simulink model "MdXX_Status"  (R2018b)
settings: Solver=FixedStepDiscrete  StartTime=0.0  StopTime=10.0  FixedStep=0.01  RelTol=1e-3
undefined symbols (not defined in the file or in its folder): data, NvStMdxxMemStatusKam_Set
libraries: RspLib x94, simulink x1
(part 2 of 2)

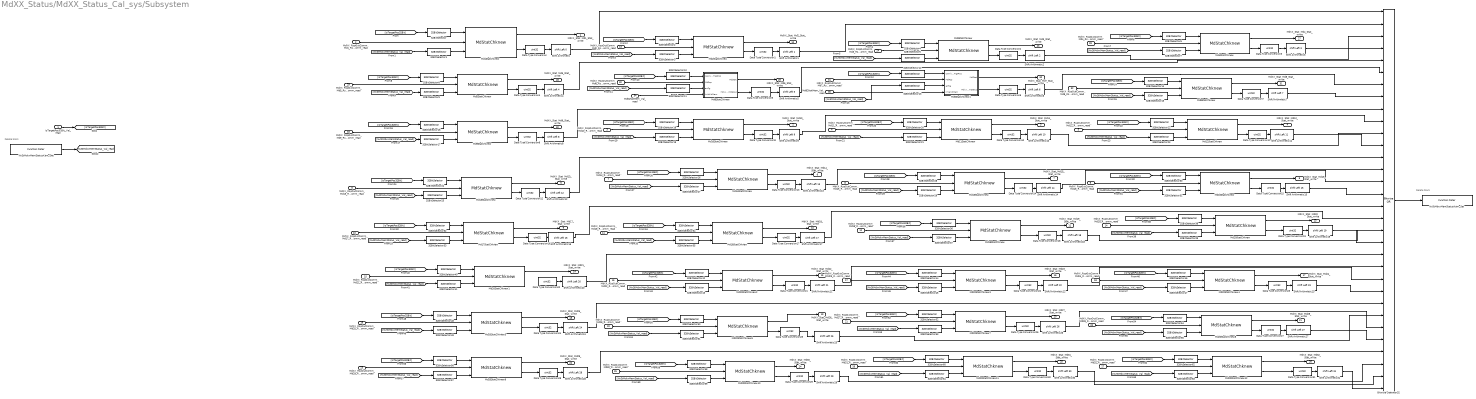
== system MdXX_Status/MdXX_Status_Cal_sys/Subsystem ==
  note: Delete block
  note: Delete block
  IsTargetPos32Bit_Val_read : Inport
  MdXX_RspOutComm_Md1_RspOutComm_read : Inport  Port=2
  MdXX_RspOutComm_Md10_RspOutComm_read : Inport  Port=3
  MdXX_RspOutComm_Md11_RspOutComm_read : Inport  Port=4
  MdXX_RspOutComm_Md12_RspOutComm_read : Inport  Port=5
  MdXX_RspOutComm_Md13_RspOutComm_read : Inport  Port=6
  MdXX_RspOutComm_Md14_RspOutComm_read : Inport  Port=7
  MdXX_RspOutComm_Md15_RspOutComm_read : Inport  Port=8
  MdXX_RspOutComm_Md16_RspOutComm_read : Inport  Port=9
  MdXX_RspOutComm_Md17_RspOutComm_read : Inport  Port=10
  MdXX_RspOutComm_Md18_RspOutComm_read : Inport  Port=11
  MdXX_RspOutComm_Md19_RspOutComm_read : Inport  Port=12
  MdXX_RspOutComm_Md2_RspOutComm_read : Inport  Port=13
  MdXX_RspOutComm_Md20_RspOutComm_read : Inport  Port=14
  MdXX_RspOutComm_Md21_RspOutComm_read : Inport  Port=15
  MdXX_RspOutComm_Md22_RspOutComm_read : Inport  Port=16
  MdXX_RspOutComm_Md23_RspOutComm_read : Inport  Port=17
  MdXX_RspOutComm_Md24_RspOutComm_read : Inport  Port=18
  MdXX_RspOutComm_Md25_RspOutComm_read : Inport  Port=19
  MdXX_RspOutComm_Md26_RspOutComm_read : Inport  Port=20
  MdXX_RspOutComm_Md27_RspOutComm_read : Inport  Port=21
  MdXX_RspOutComm_Md28_RspOutComm_read : Inport  Port=22
  MdXX_RspOutComm_Md29_RspOutComm_read : Inport  Port=23
  MdXX_RspOutComm_Md3_RspOutComm_read : Inport  Port=24
  MdXX_RspOutComm_Md30_RspOutComm_read : Inport  Port=25
  MdXX_RspOutComm_Md31_RspOutComm_read : Inport  Port=26
  MdXX_RspOutComm_Md32_RspOutComm_read : Inport  Port=27
  MdXX_RspOutComm_Md4_RspOutComm_read : Inport  Port=28
  MdXX_RspOutComm_Md5_RspOutComm_read : Inport  Port=29
  MdXX_RspOutComm_Md6_RspOutComm_read : Inport  Port=30
  MdXX_RspOutComm_Md7_RspOutComm_read : Inport  Port=31
  MdXX_RspOutComm_Md8_RspOutComm_read : Inport  Port=32
  MdXX_RspOutComm_Md9_RspOutComm_read : Inport  Port=33
  Md61NotMem_Val_read : Inport  Port=34
  Md62NotMem_Val_read : Inport  Port=35
  32BitSelector : RspLib/32BitSelector  BitNum=0
  32BitSelector1 : RspLib/32BitSelector  BitNum=0
  32BitSelector10 : RspLib/32BitSelector  BitNum=5
  32BitSelector11 : RspLib/32BitSelector  BitNum=5
  32BitSelector12 : RspLib/32BitSelector  BitNum=6
  32BitSelector13 : RspLib/32BitSelector  BitNum=6
  32BitSelector14 : RspLib/32BitSelector  BitNum=7
  32BitSelector15 : RspLib/32BitSelector  BitNum=7
  32BitSelector16 : RspLib/32BitSelector  BitNum=8
  32BitSelector17 : RspLib/32BitSelector  BitNum=8
  32BitSelector18 : RspLib/32BitSelector  BitNum=9
  32BitSelector19 : RspLib/32BitSelector  BitNum=9
  32BitSelector2 : RspLib/32BitSelector  BitNum=1
  32BitSelector20 : RspLib/32BitSelector  BitNum=10
  32BitSelector21 : RspLib/32BitSelector  BitNum=10
  32BitSelector22 : RspLib/32BitSelector  BitNum=11
  32BitSelector23 : RspLib/32BitSelector  BitNum=11
  32BitSelector24 : RspLib/32BitSelector  BitNum=12
  32BitSelector25 : RspLib/32BitSelector  BitNum=12
  32BitSelector26 : RspLib/32BitSelector  BitNum=13
  32BitSelector27 : RspLib/32BitSelector  BitNum=13
  32BitSelector28 : RspLib/32BitSelector  BitNum=14
  32BitSelector29 : RspLib/32BitSelector  BitNum=14
  32BitSelector3 : RspLib/32BitSelector  BitNum=1
  32BitSelector30 : RspLib/32BitSelector  BitNum=15
  32BitSelector31 : RspLib/32BitSelector  BitNum=15
  32BitSelector32 : RspLib/32BitSelector  BitNum=16
  32BitSelector33 : RspLib/32BitSelector  BitNum=16
  32BitSelector34 : RspLib/32BitSelector  BitNum=17
  32BitSelector35 : RspLib/32BitSelector  BitNum=17
  32BitSelector36 : RspLib/32BitSelector  BitNum=18
  32BitSelector37 : RspLib/32BitSelector  BitNum=18
  32BitSelector38 : RspLib/32BitSelector  BitNum=19
  32BitSelector39 : RspLib/32BitSelector  BitNum=19
  32BitSelector4 : RspLib/32BitSelector  BitNum=2
  32BitSelector40 : RspLib/32BitSelector  BitNum=20
  32BitSelector41 : RspLib/32BitSelector  BitNum=20
  32BitSelector42 : RspLib/32BitSelector  BitNum=21
  32BitSelector43 : RspLib/32BitSelector  BitNum=21
  32BitSelector44 : RspLib/32BitSelector  BitNum=22
  32BitSelector45 : RspLib/32BitSelector  BitNum=22
  32BitSelector46 : RspLib/32BitSelector  BitNum=23
  32BitSelector47 : RspLib/32BitSelector  BitNum=23
  32BitSelector48 : RspLib/32BitSelector  BitNum=24
  32BitSelector49 : RspLib/32BitSelector  BitNum=24
  32BitSelector5 : RspLib/32BitSelector  BitNum=2
  32BitSelector50 : RspLib/32BitSelector  BitNum=25
  32BitSelector51 : RspLib/32BitSelector  BitNum=25
  32BitSelector52 : RspLib/32BitSelector  BitNum=26
  32BitSelector53 : RspLib/32BitSelector  BitNum=26
  32BitSelector54 : RspLib/32BitSelector  BitNum=27
  32BitSelector55 : RspLib/32BitSelector  BitNum=27
  32BitSelector56 : RspLib/32BitSelector  BitNum=28
  32BitSelector57 : RspLib/32BitSelector  BitNum=28
  32BitSelector58 : RspLib/32BitSelector  BitNum=29
  32BitSelector59 : RspLib/32BitSelector  BitNum=29
  32BitSelector6 : RspLib/32BitSelector  BitNum=3
  32BitSelector60 : RspLib/32BitSelector  BitNum=30
  32BitSelector61 : RspLib/32BitSelector  BitNum=30
  32BitSelector62 : RspLib/32BitSelector  BitNum=31
  32BitSelector63 : RspLib/32BitSelector  BitNum=31
  32BitSelector7 : RspLib/32BitSelector  BitNum=3
  32BitSelector8 : RspLib/32BitSelector  BitNum=4
  32BitSelector9 : RspLib/32BitSelector  BitNum=4
  Bitwise Operator32 : simulink/Logic and Bit Operations/Bitwise Operator  logicop=OR  UseBitMask=off  NumInputPorts=32  BitMask=bin2dec('11011001')  BitMaskRealWorld=Stored Integer
  Data Type Conversion{,1..31} (32 alike) : DataTypeConversion  OutDataTypeStr=uint32
  Md10StatChknew : RspLib/MdStatChknew  SystemSampleTime=-1
  Md11StatChknew : RspLib/MdStatChknew  SystemSampleTime=-1
  Md12StatChknew : RspLib/MdStatChknew  SystemSampleTime=-1
  Md13StatChknew : RspLib/MdStatChknew  SystemSampleTime=-1
  Md14StatChknew : RspLib/MdStatChknew  SystemSampleTime=-1
  Md15StatChknew : RspLib/MdStatChknew  SystemSampleTime=-1
  Md16StatChknew : RspLib/MdStatChknew  SystemSampleTime=-1
  Md17StatChknew : RspLib/MdStatChknew  SystemSampleTime=-1
  Md18StatChknew : RspLib/MdStatChknew  SystemSampleTime=-1
  Md19StatChknew : RspLib/MdStatChknew  SystemSampleTime=-1
  Md1StatChknew : RspLib/MdStatChknew  SystemSampleTime=-1
  Md20StatChknew{,1..12} (13 alike) : RspLib/MdStatChknew  SystemSampleTime=-1
  Md2StatChknew : RspLib/MdStatChknew  SystemSampleTime=-1
  Md3StatChknew : RspLib/MdStatChknew  SystemSampleTime=-1
  Md4StatChknew : RspLib/MdStatChknew  SystemSampleTime=-1
  Md5StatChknew : RspLib/MdStatChknew  SystemSampleTime=-1
  Md6StatChknew : Subsystem
  Md6StatChknew1 : Subsystem
  Md8StatChknew : RspLib/MdStatChknew  SystemSampleTime=-1
  Md9StatChknew : RspLib/MdStatChknew  SystemSampleTime=-1
  NvStMdxxMemStatusKam_Get : FunctionCaller  FunctionPrototype=data = NvStMdxxMemStatusKam_Get()  OutputArgumentSpecifications=uint32(1)
  NvStMdxxMemStatusKam_Set : FunctionCaller  FunctionPrototype=NvStMdxxMemStatusKam_Set(data)  InputArgumentSpecifications=uint32(1)
  Shift Arithmetic : ArithShift  BitShiftDirection=Left
  Shift Arithmetic1 : ArithShift  BitShiftNumber=1  BitShiftDirection=Left
  Shift Arithmetic10 : ArithShift  BitShiftNumber=10  BitShiftDirection=Left
  Shift Arithmetic11 : ArithShift  BitShiftNumber=11  BitShiftDirection=Left
  Shift Arithmetic12 : ArithShift  BitShiftNumber=12  BitShiftDirection=Left
  Shift Arithmetic13 : ArithShift  BitShiftNumber=13  BitShiftDirection=Left
  Shift Arithmetic14 : ArithShift  BitShiftNumber=14  BitShiftDirection=Left
  Shift Arithmetic15 : ArithShift  BitShiftNumber=15  BitShiftDirection=Left
  Shift Arithmetic16 : ArithShift  BitShiftNumber=16  BitShiftDirection=Left
  Shift Arithmetic17 : ArithShift  BitShiftNumber=17  BitShiftDirection=Left
  Shift Arithmetic18 : ArithShift  BitShiftNumber=18  BitShiftDirection=Left
  Shift Arithmetic19 : ArithShift  BitShiftNumber=19  BitShiftDirection=Left
  Shift Arithmetic2 : ArithShift  BitShiftNumber=2  BitShiftDirection=Left
  Shift Arithmetic20 : ArithShift  BitShiftNumber=20  BitShiftDirection=Left
  Shift Arithmetic21 : ArithShift  BitShiftNumber=21  BitShiftDirection=Left
  Shift Arithmetic22 : ArithShift  BitShiftNumber=22  BitShiftDirection=Left
  Shift Arithmetic23 : ArithShift  BitShiftNumber=23  BitShiftDirection=Left
  Shift Arithmetic24 : ArithShift  BitShiftNumber=24  BitShiftDirection=Left
  Shift Arithmetic25 : ArithShift  BitShiftNumber=25  BitShiftDirection=Left
  Shift Arithmetic26 : ArithShift  BitShiftNumber=26  BitShiftDirection=Left
  Shift Arithmetic27 : ArithShift  BitShiftNumber=27  BitShiftDirection=Left
  Shift Arithmetic28 : ArithShift  BitShiftNumber=28  BitShiftDirection=Left
  Shift Arithmetic29 : ArithShift  BitShiftNumber=29  BitShiftDirection=Left
  Shift Arithmetic3 : ArithShift  BitShiftNumber=3  BitShiftDirection=Left
  Shift Arithmetic30 : ArithShift  BitShiftNumber=30  BitShiftDirection=Left
  Shift Arithmetic31 : ArithShift  BitShiftNumber=31  BitShiftDirection=Left
  Shift Arithmetic4 : ArithShift  BitShiftNumber=4  BitShiftDirection=Left
  Shift Arithmetic5 : ArithShift  BitShiftNumber=5  BitShiftDirection=Left
  Shift Arithmetic6 : ArithShift  BitShiftNumber=6  BitShiftDirection=Left
  Shift Arithmetic7 : ArithShift  BitShiftNumber=7  BitShiftDirection=Left
  Shift Arithmetic8 : ArithShift  BitShiftNumber=8  BitShiftDirection=Left
  Shift Arithmetic9 : ArithShift  BitShiftNumber=9  BitShiftDirection=Left
  MdXX_Stat_Md1_Stat_write : Outport
      settings: EnsureOutportIsVirtual=on
  MdXX_Stat_Md10_Stat_write : Outport  Port=2
      settings: EnsureOutportIsVirtual=on
  MdXX_Stat_Md11_Stat_write : Outport  Port=3
      settings: EnsureOutportIsVirtual=on
  MdXX_Stat_Md12_Stat_write : Outport  Port=4
      settings: EnsureOutportIsVirtual=on
  MdXX_Stat_Md13_Stat_write : Outport  Port=5
      settings: EnsureOutportIsVirtual=on
  MdXX_Stat_Md14_Stat_write : Outport  Port=6
      settings: EnsureOutportIsVirtual=on
  MdXX_Stat_Md15_Stat_write : Outport  Port=7
      settings: EnsureOutportIsVirtual=on
  MdXX_Stat_Md16_Stat_write : Outport  Port=8
      settings: EnsureOutportIsVirtual=on
  MdXX_Stat_Md17_Stat_write : Outport  Port=9
      settings: EnsureOutportIsVirtual=on
  MdXX_Stat_Md18_Stat_write : Outport  Port=10
      settings: EnsureOutportIsVirtual=on
  MdXX_Stat_Md19_Stat_write : Outport  Port=11
      settings: EnsureOutportIsVirtual=on
  MdXX_Stat_Md2_Stat_write : Outport  Port=12
      settings: EnsureOutportIsVirtual=on
  MdXX_Stat_Md20_Stat_write : Outport  Port=13
      settings: EnsureOutportIsVirtual=on
  MdXX_Stat_Md21_Stat_write : Outport  Port=14
      settings: EnsureOutportIsVirtual=on
  MdXX_Stat_Md22_Stat_write : Outport  Port=15
      settings: EnsureOutportIsVirtual=on
  MdXX_Stat_Md23_Stat_write : Outport  Port=16
      settings: EnsureOutportIsVirtual=on
  MdXX_Stat_Md24_Stat_write : Outport  Port=17
      settings: EnsureOutportIsVirtual=on
  MdXX_Stat_Md25_Stat_write : Outport  Port=18
      settings: EnsureOutportIsVirtual=on
  MdXX_Stat_Md26_Stat_write : Outport  Port=19
      settings: EnsureOutportIsVirtual=on
  MdXX_Stat_Md27_Stat_write : Outport  Port=20
      settings: EnsureOutportIsVirtual=on
  MdXX_Stat_Md28_Stat_write : Outport  Port=21
      settings: EnsureOutportIsVirtual=on
  MdXX_Stat_Md29_Stat_write : Outport  Port=22
      settings: EnsureOutportIsVirtual=on
  MdXX_Stat_Md3_Stat_write : Outport  Port=23
      settings: EnsureOutportIsVirtual=on
  MdXX_Stat_Md30_Stat_write : Outport  Port=24
      settings: EnsureOutportIsVirtual=on
  MdXX_Stat_Md31_Stat_write : Outport  Port=25
      settings: EnsureOutportIsVirtual=on
  MdXX_Stat_Md32_Stat_write : Outport  Port=26
      settings: EnsureOutportIsVirtual=on
  MdXX_Stat_Md4_Stat_write : Outport  Port=27
      settings: EnsureOutportIsVirtual=on
  MdXX_Stat_Md5_Stat_write : Outport  Port=28
      settings: EnsureOutportIsVirtual=on
  MdXX_Stat_Md6_Stat_write : Outport  Port=29
      settings: EnsureOutportIsVirtual=on
  MdXX_Stat_Md7_Stat_write : Outport  Port=30
      settings: EnsureOutportIsVirtual=on
  MdXX_Stat_Md8_Stat_write : Outport  Port=31
      settings: EnsureOutportIsVirtual=on
  MdXX_Stat_Md9_Stat_write : Outport  Port=32
      settings: EnsureOutportIsVirtual=on
  wires:
  IsTargetPos32Bit_Val_read/1 -> [IsTargetPos32Bit]
  [IsTargetPos32Bit] -> 32BitSelector/1
  32BitSelector/1 -> Md1StatChknew/1
  32BitSelector1/1 -> Md1StatChknew/3
  MdXX_RspOutComm_Md1_RspOutComm_read/1 -> Md1StatChknew/2
  MdXX_RspOutComm_Md2_RspOutComm_read/1 -> Md2StatChknew/2
  32BitSelector3/1 -> Md2StatChknew/3
  32BitSelector2/1 -> Md2StatChknew/1
  [IsTargetPos32Bit] -> 32BitSelector2/1
  [NvStMdxxMemStatus_Val_read] -> 32BitSelector5/1
  [IsTargetPos32Bit] -> 32BitSelector4/1
  32BitSelector4/1 -> Md3StatChknew/1
  32BitSelector5/1 -> Md3StatChknew/3
  MdXX_RspOutComm_Md3_RspOutComm_read/1 -> Md3StatChknew/2
  MdXX_RspOutComm_Md4_RspOutComm_read/1 -> Md4StatChknew/2
  32BitSelector7/1 -> Md4StatChknew/3
  32BitSelector6/1 -> Md4StatChknew/1
  [IsTargetPos32Bit] -> 32BitSelector6/1
  [NvStMdxxMemStatus_Val_read] -> 32BitSelector7/1
  [IsTargetPos32Bit] -> 32BitSelector8/1
  32BitSelector8/1 -> Md5StatChknew/1
  32BitSelector9/1 -> Md5StatChknew/3
  MdXX_RspOutComm_Md5_RspOutComm_read/1 -> Md5StatChknew/2
  MdXX_RspOutComm_Md6_RspOutComm_read/1 -> Md6StatChknew/2(MdRsp)
  32BitSelector11/1 -> Md6StatChknew/3(enflg)
  32BitSelector10/1 -> Md6StatChknew/1(IsArrivedTrgtPos)
  [IsTargetPos32Bit] -> 32BitSelector10/1
  [NvStMdxxMemStatus_Val_read] -> 32BitSelector11/1
  [IsTargetPos32Bit] -> 32BitSelector12/1
  32BitSelector12/1 -> Md6StatChknew1/1(IsArrivedTrgtPos)
  32BitSelector13/1 -> Md6StatChknew1/3(enflg)
  MdXX_RspOutComm_Md7_RspOutComm_read/1 -> Md6StatChknew1/2(MdRsp)
  MdXX_RspOutComm_Md8_RspOutComm_read/1 -> Md8StatChknew/2
  32BitSelector15/1 -> Md8StatChknew/3
  32BitSelector14/1 -> Md8StatChknew/1
  [IsTargetPos32Bit] -> 32BitSelector14/1
  [IsTargetPos32Bit] -> 32BitSelector16/1
  32BitSelector16/1 -> Md9StatChknew/1
  32BitSelector17/1 -> Md9StatChknew/3
  MdXX_RspOutComm_Md9_RspOutComm_read/1 -> Md9StatChknew/2
  MdXX_RspOutComm_Md10_RspOutComm_read/1 -> Md10StatChknew/2
  32BitSelector19/1 -> Md10StatChknew/3
  32BitSelector18/1 -> Md10StatChknew/1
  [IsTargetPos32Bit] -> 32BitSelector18/1
  [IsTargetPos32Bit] -> 32BitSelector20/1
  32BitSelector20/1 -> Md11StatChknew/1
  32BitSelector21/1 -> Md11StatChknew/3
  MdXX_RspOutComm_Md11_RspOutComm_read/1 -> Md11StatChknew/2
  MdXX_RspOutComm_Md12_RspOutComm_read/1 -> Md12StatChknew/2
  32BitSelector23/1 -> Md12StatChknew/3
  32BitSelector22/1 -> Md12StatChknew/1
  [IsTargetPos32Bit] -> 32BitSelector22/1
  [IsTargetPos32Bit] -> 32BitSelector24/1
  32BitSelector24/1 -> Md13StatChknew/1
  32BitSelector25/1 -> Md13StatChknew/3
  MdXX_RspOutComm_Md13_RspOutComm_read/1 -> Md13StatChknew/2
  MdXX_RspOutComm_Md14_RspOutComm_read/1 -> Md14StatChknew/2
  32BitSelector27/1 -> Md14StatChknew/3
  32BitSelector26/1 -> Md14StatChknew/1
  [IsTargetPos32Bit] -> 32BitSelector26/1
  [IsTargetPos32Bit] -> 32BitSelector28/1
  32BitSelector28/1 -> Md15StatChknew/1
  32BitSelector29/1 -> Md15StatChknew/3
  MdXX_RspOutComm_Md15_RspOutComm_read/1 -> Md15StatChknew/2
  MdXX_RspOutComm_Md16_RspOutComm_read/1 -> Md16StatChknew/2
  32BitSelector31/1 -> Md16StatChknew/3
  32BitSelector30/1 -> Md16StatChknew/1
  [IsTargetPos32Bit] -> 32BitSelector30/1
  [IsTargetPos32Bit] -> 32BitSelector32/1
  32BitSelector32/1 -> Md17StatChknew/1
  32BitSelector33/1 -> Md17StatChknew/3
  MdXX_RspOutComm_Md17_RspOutComm_read/1 -> Md17StatChknew/2
  MdXX_RspOutComm_Md18_RspOutComm_read/1 -> Md18StatChknew/2
  32BitSelector35/1 -> Md18StatChknew/3
  32BitSelector34/1 -> Md18StatChknew/1
  [IsTargetPos32Bit] -> 32BitSelector34/1
  [IsTargetPos32Bit] -> 32BitSelector36/1
  32BitSelector36/1 -> Md19StatChknew/1
  32BitSelector37/1 -> Md19StatChknew/3
  MdXX_RspOutComm_Md19_RspOutComm_read/1 -> Md19StatChknew/2
  MdXX_RspOutComm_Md20_RspOutComm_read/1 -> Md20StatChknew/2
  32BitSelector39/1 -> Md20StatChknew/3
  32BitSelector38/1 -> Md20StatChknew/1
  [IsTargetPos32Bit] -> 32BitSelector38/1
  Md1StatChknew/1 -> MdXX_Stat_Md1_Stat_write/1
  Md2StatChknew/1 -> MdXX_Stat_Md2_Stat_write/1
  Md3StatChknew/1 -> MdXX_Stat_Md3_Stat_write/1
  Md4StatChknew/1 -> MdXX_Stat_Md4_Stat_write/1
  Md5StatChknew/1 -> MdXX_Stat_Md5_Stat_write/1
  Md6StatChknew/1(MdStat) -> MdXX_Stat_Md6_Stat_write/1
  Md6StatChknew1/1(MdStat) -> MdXX_Stat_Md7_Stat_write/1
  Md8StatChknew/1 -> MdXX_Stat_Md8_Stat_write/1
  Md9StatChknew/1 -> MdXX_Stat_Md9_Stat_write/1
  Md10StatChknew/1 -> MdXX_Stat_Md10_Stat_write/1
  Md11StatChknew/1 -> MdXX_Stat_Md11_Stat_write/1
  Md12StatChknew/1 -> MdXX_Stat_Md12_Stat_write/1
  Md13StatChknew/1 -> MdXX_Stat_Md13_Stat_write/1
  Md14StatChknew/1 -> MdXX_Stat_Md14_Stat_write/1
  Md15StatChknew/1 -> MdXX_Stat_Md15_Stat_write/1
  Md16StatChknew/1 -> MdXX_Stat_Md16_Stat_write/1
  Md17StatChknew/1 -> MdXX_Stat_Md17_Stat_write/1
  Md18StatChknew/1 -> MdXX_Stat_Md18_Stat_write/1
  Md19StatChknew/1 -> MdXX_Stat_Md19_Stat_write/1
  Md20StatChknew/1 -> MdXX_Stat_Md20_Stat_write/1
  Md20StatChknew1/1 -> MdXX_Stat_Md21_Stat_write/1
  [IsTargetPos32Bit] -> 32BitSelector40/1
  32BitSelector40/1 -> Md20StatChknew1/1
  32BitSelector41/1 -> Md20StatChknew1/3
  MdXX_RspOutComm_Md21_RspOutComm_read/1 -> Md20StatChknew1/2
  MdXX_RspOutComm_Md22_RspOutComm_read/1 -> Md20StatChknew2/2
  32BitSelector43/1 -> Md20StatChknew2/3
  32BitSelector42/1 -> Md20StatChknew2/1
  [IsTargetPos32Bit] -> 32BitSelector42/1
  Md20StatChknew2/1 -> MdXX_Stat_Md22_Stat_write/1
  Md20StatChknew3/1 -> MdXX_Stat_Md23_Stat_write/1
  [IsTargetPos32Bit] -> 32BitSelector44/1
  32BitSelector44/1 -> Md20StatChknew3/1
  32BitSelector45/1 -> Md20StatChknew3/3
  MdXX_RspOutComm_Md23_RspOutComm_read/1 -> Md20StatChknew3/2
  MdXX_RspOutComm_Md24_RspOutComm_read/1 -> Md20StatChknew4/2
  32BitSelector47/1 -> Md20StatChknew4/3
  32BitSelector46/1 -> Md20StatChknew4/1
  [IsTargetPos32Bit] -> 32BitSelector46/1
  Md20StatChknew4/1 -> MdXX_Stat_Md24_Stat_write/1
  Md20StatChknew5/1 -> MdXX_Stat_Md25_Stat_write/1
  [IsTargetPos32Bit] -> 32BitSelector48/1
  32BitSelector48/1 -> Md20StatChknew5/1
  32BitSelector49/1 -> Md20StatChknew5/3
  MdXX_RspOutComm_Md25_RspOutComm_read/1 -> Md20StatChknew5/2
  MdXX_RspOutComm_Md26_RspOutComm_read/1 -> Md20StatChknew6/2
  32BitSelector51/1 -> Md20StatChknew6/3
  32BitSelector50/1 -> Md20StatChknew6/1
  [IsTargetPos32Bit] -> 32BitSelector50/1
  Md20StatChknew6/1 -> MdXX_Stat_Md26_Stat_write/1
  Md20StatChknew7/1 -> MdXX_Stat_Md27_Stat_write/1
  [IsTargetPos32Bit] -> 32BitSelector52/1
  32BitSelector52/1 -> Md20StatChknew7/1
  32BitSelector53/1 -> Md20StatChknew7/3
  MdXX_RspOutComm_Md27_RspOutComm_read/1 -> Md20StatChknew7/2
  MdXX_RspOutComm_Md28_RspOutComm_read/1 -> Md20StatChknew8/2
  32BitSelector55/1 -> Md20StatChknew8/3
  32BitSelector54/1 -> Md20StatChknew8/1
  [IsTargetPos32Bit] -> 32BitSelector54/1
  Md20StatChknew8/1 -> MdXX_Stat_Md28_Stat_write/1
  Md20StatChknew9/1 -> MdXX_Stat_Md29_Stat_write/1
  [IsTargetPos32Bit] -> 32BitSelector56/1
  32BitSelector56/1 -> Md20StatChknew9/1
  32BitSelector57/1 -> Md20StatChknew9/3
  MdXX_RspOutComm_Md29_RspOutComm_read/1 -> Md20StatChknew9/2
  MdXX_RspOutComm_Md30_RspOutComm_read/1 -> Md20StatChknew10/2
  32BitSelector59/1 -> Md20StatChknew10/3
  32BitSelector58/1 -> Md20StatChknew10/1
  [IsTargetPos32Bit] -> 32BitSelector58/1
  Md20StatChknew10/1 -> MdXX_Stat_Md30_Stat_write/1
  Md20StatChknew11/1 -> MdXX_Stat_Md31_Stat_write/1
  [IsTargetPos32Bit] -> 32BitSelector60/1
  32BitSelector60/1 -> Md20StatChknew11/1
  32BitSelector61/1 -> Md20StatChknew11/3
  MdXX_RspOutComm_Md31_RspOutComm_read/1 -> Md20StatChknew11/2
  MdXX_RspOutComm_Md32_RspOutComm_read/1 -> Md20StatChknew12/2
  32BitSelector63/1 -> Md20StatChknew12/3
  32BitSelector62/1 -> Md20StatChknew12/1
  [IsTargetPos32Bit] -> 32BitSelector62/1
  Md20StatChknew12/1 -> MdXX_Stat_Md32_Stat_write/1
  Md61NotMem_Val_read/1 -> Md6StatChknew/4(InValidMem)
  Md62NotMem_Val_read/1 -> Md6StatChknew1/4(InValidMem)
  Data Type Conversion/1 -> Shift Arithmetic/1
  Md1StatChknew/2 -> Data Type Conversion/1
  Shift Arithmetic/1 -> Bitwise Operator32/1
  [NvStMdxxMemStatus_Val_read] -> 32BitSelector1/1
  Md2StatChknew/2 -> Data Type Conversion1/1
  [NvStMdxxMemStatus_Val_read] -> 32BitSelector3/1
  Data Type Conversion1/1 -> Shift Arithmetic1/1
  Shift Arithmetic1/1 -> Bitwise Operator32/2
  Md3StatChknew/2 -> Data Type Conversion2/1
  Data Type Conversion2/1 -> Shift Arithmetic2/1
  Shift Arithmetic2/1 -> Bitwise Operator32/3
  Md4StatChknew/2 -> Data Type Conversion3/1
  Data Type Conversion3/1 -> Shift Arithmetic3/1
  Shift Arithmetic3/1 -> Bitwise Operator32/4
  Md5StatChknew/2 -> Data Type Conversion4/1
  Data Type Conversion4/1 -> Shift Arithmetic4/1
  Shift Arithmetic4/1 -> Bitwise Operator32/5
  Md6StatChknew/2(MdxxMemStatus) -> Data Type Conversion5/1
  Data Type Conversion5/1 -> Shift Arithmetic5/1
  Md6StatChknew1/2(MdxxMemStatus) -> Data Type Conversion6/1
  [NvStMdxxMemStatus_Val_read] -> 32BitSelector13/1
  Data Type Conversion6/1 -> Shift Arithmetic6/1
  Md8StatChknew/2 -> Data Type Conversion7/1
  Data Type Conversion7/1 -> Shift Arithmetic7/1
  Shift Arithmetic7/1 -> Bitwise Operator32/8
  Md9StatChknew/2 -> Data Type Conversion8/1
  Data Type Conversion8/1 -> Shift Arithmetic8/1
  Shift Arithmetic8/1 -> Bitwise Operator32/9
  Md10StatChknew/2 -> Data Type Conversion9/1
  Data Type Conversion9/1 -> Shift Arithmetic9/1
  Shift Arithmetic9/1 -> Bitwise Operator32/10
  Md11StatChknew/2 -> Data Type Conversion10/1
  Data Type Conversion10/1 -> Shift Arithmetic10/1
  Shift Arithmetic10/1 -> Bitwise Operator32/11
  [NvStMdxxMemStatus_Val_read] -> 32BitSelector21/1
  Md12StatChknew/2 -> Data Type Conversion11/1
  Data Type Conversion11/1 -> Shift Arithmetic11/1
  Shift Arithmetic11/1 -> Bitwise Operator32/12
  Md13StatChknew/2 -> Data Type Conversion12/1
  Data Type Conversion12/1 -> Shift Arithmetic12/1
  Shift Arithmetic12/1 -> Bitwise Operator32/13
  Md14StatChknew/2 -> Data Type Conversion13/1
  Data Type Conversion13/1 -> Shift Arithmetic13/1
  Shift Arithmetic13/1 -> Bitwise Operator32/14
  Shift Arithmetic14/1 -> Bitwise Operator32/15
  Data Type Conversion14/1 -> Shift Arithmetic14/1
  Md15StatChknew/2 -> Data Type Conversion14/1
  Shift Arithmetic15/1 -> Bitwise Operator32/16
  Data Type Conversion15/1 -> Shift Arithmetic15/1
  Md16StatChknew/2 -> Data Type Conversion15/1
  Shift Arithmetic16/1 -> Bitwise Operator32/17
  Data Type Conversion16/1 -> Shift Arithmetic16/1
  Md17StatChknew/2 -> Data Type Conversion16/1
  Shift Arithmetic17/1 -> Bitwise Operator32/18
  Data Type Conversion17/1 -> Shift Arithmetic17/1
  Md18StatChknew/2 -> Data Type Conversion17/1
  Shift Arithmetic18/1 -> Bitwise Operator32/19
  Data Type Conversion18/1 -> Shift Arithmetic18/1
  Md19StatChknew/2 -> Data Type Conversion18/1
  Shift Arithmetic19/1 -> Bitwise Operator32/20
  Data Type Conversion19/1 -> Shift Arithmetic19/1
  Md20StatChknew/2 -> Data Type Conversion19/1
  Shift Arithmetic20/1 -> Bitwise Operator32/21
  Data Type Conversion20/1 -> Shift Arithmetic20/1
  ? -> Data Type Conversion20/1
  Shift Arithmetic21/1 -> Bitwise Operator32/22
  Data Type Conversion21/1 -> Shift Arithmetic21/1
  Md20StatChknew2/2 -> Data Type Conversion21/1
  Shift Arithmetic22/1 -> Bitwise Operator32/23
  Data Type Conversion22/1 -> Shift Arithmetic22/1
  Md20StatChknew3/2 -> Data Type Conversion22/1
  Shift Arithmetic23/1 -> Bitwise Operator32/24
  Data Type Conversion23/1 -> Shift Arithmetic23/1
  [NvStMdxxMemStatus_Val_read] -> 32BitSelector47/1
  Md20StatChknew4/2 -> Data Type Conversion23/1
  Shift Arithmetic24/1 -> Bitwise Operator32/25
  Data Type Conversion24/1 -> Shift Arithmetic24/1
  Md20StatChknew5/2 -> Data Type Conversion24/1
  Shift Arithmetic25/1 -> Bitwise Operator32/26
  Data Type Conversion25/1 -> Shift Arithmetic25/1
  Md20StatChknew6/2 -> Data Type Conversion25/1
  Shift Arithmetic26/1 -> Bitwise Operator32/27
  Data Type Conversion26/1 -> Shift Arithmetic26/1
  Md20StatChknew7/2 -> Data Type Conversion26/1
  Shift Arithmetic27/1 -> Bitwise Operator32/28
  Data Type Conversion27/1 -> Shift Arithmetic27/1
  Md20StatChknew8/2 -> Data Type Conversion27/1
  Data Type Conversion28/1 -> Shift Arithmetic28/1
  Md20StatChknew9/2 -> Data Type Conversion28/1
  Shift Arithmetic29/1 -> Bitwise Operator32/30
  Data Type Conversion29/1 -> Shift Arithmetic29/1
  Md20StatChknew10/2 -> Data Type Conversion29/1
  Data Type Conversion30/1 -> Shift Arithmetic30/1
  Md20StatChknew11/2 -> Data Type Conversion30/1
  Data Type Conversion31/1 -> Shift Arithmetic31/1
  Md20StatChknew12/2 -> Data Type Conversion31/1
  NvStMdxxMemStatusKam_Get/1 -> [NvStMdxxMemStatus_Val_read]
  [NvStMdxxMemStatus_Val_read] -> 32BitSelector9/1
  [NvStMdxxMemStatus_Val_read] -> 32BitSelector15/1
  [NvStMdxxMemStatus_Val_read] -> 32BitSelector17/1
  [NvStMdxxMemStatus_Val_read] -> 32BitSelector19/1
  [NvStMdxxMemStatus_Val_read] -> 32BitSelector23/1
  [NvStMdxxMemStatus_Val_read] -> 32BitSelector25/1
  [NvStMdxxMemStatus_Val_read] -> 32BitSelector27/1
  [NvStMdxxMemStatus_Val_read] -> 32BitSelector29/1
  [NvStMdxxMemStatus_Val_read] -> 32BitSelector31/1
  [NvStMdxxMemStatus_Val_read] -> 32BitSelector33/1
  [NvStMdxxMemStatus_Val_read] -> 32BitSelector35/1
  [NvStMdxxMemStatus_Val_read] -> 32BitSelector37/1
  [NvStMdxxMemStatus_Val_read] -> 32BitSelector39/1
  [NvStMdxxMemStatus_Val_read] -> 32BitSelector41/1
  [NvStMdxxMemStatus_Val_read] -> 32BitSelector43/1
  [NvStMdxxMemStatus_Val_read] -> 32BitSelector45/1
  [NvStMdxxMemStatus_Val_read] -> 32BitSelector49/1
  [NvStMdxxMemStatus_Val_read] -> 32BitSelector51/1
  [NvStMdxxMemStatus_Val_read] -> 32BitSelector53/1
  [NvStMdxxMemStatus_Val_read] -> 32BitSelector55/1
  [NvStMdxxMemStatus_Val_read] -> 32BitSelector57/1
  [NvStMdxxMemStatus_Val_read] -> 32BitSelector59/1
  [NvStMdxxMemStatus_Val_read] -> 32BitSelector61/1
  [NvStMdxxMemStatus_Val_read] -> 32BitSelector63/1
  Shift Arithmetic5/1 -> Bitwise Operator32/6
  Shift Arithmetic6/1 -> Bitwise Operator32/7
  Shift Arithmetic28/1 -> Bitwise Operator32/29
  Shift Arithmetic30/1 -> Bitwise Operator32/31
  Shift Arithmetic31/1 -> Bitwise Operator32/32
  Bitwise Operator32/1 -> NvStMdxxMemStatusKam_Set/1

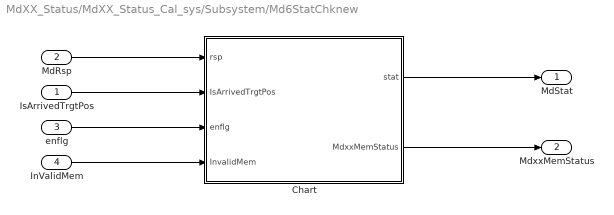
== system MdXX_Status/MdXX_Status_Cal_sys/Subsystem/Md6StatChknew ==
  IsArrivedTrgtPos : Inport
  MdRsp : Inport  Port=2
  enflg : Inport  Port=3
  InValidMem : Inport  Port=4
  Chart : Stateflow chart  TreatAsAtomicUnit=on
      settings: RTWSystemCode=Inline
  MdStat : Outport
  MdxxMemStatus : Outport  Port=2
  wires:
  Chart/1(stat) -> MdStat/1
  IsArrivedTrgtPos/1 -> Chart/2(IsArrivedTrgtPos)
  enflg/1 -> Chart/3(enflg)
  MdRsp/1 -> Chart/1(rsp)
  InValidMem/1 -> Chart/4(InvalidMem)
  Chart/2(MdxxMemStatus) -> MdxxMemStatus/1

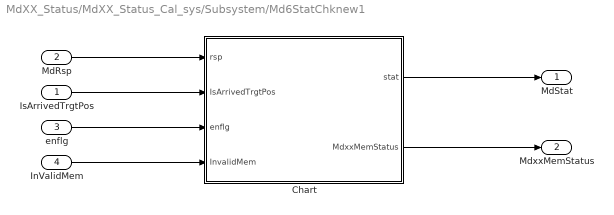
== system MdXX_Status/MdXX_Status_Cal_sys/Subsystem/Md6StatChknew1 ==
  IsArrivedTrgtPos : Inport
  MdRsp : Inport  Port=2
  enflg : Inport  Port=3
  InValidMem : Inport  Port=4
  Chart : Stateflow chart  TreatAsAtomicUnit=on
      settings: RTWSystemCode=Inline
  MdStat : Outport
  MdxxMemStatus : Outport  Port=2
  wires:
  Chart/1(stat) -> MdStat/1
  IsArrivedTrgtPos/1 -> Chart/2(IsArrivedTrgtPos)
  enflg/1 -> Chart/3(enflg)
  MdRsp/1 -> Chart/1(rsp)
  InValidMem/1 -> Chart/4(InvalidMem)
  Chart/2(MdxxMemStatus) -> MdxxMemStatus/1

== stateflow chart MdXX_Status/MdXX_Status_Cal_sys/Subsystem/Md6StatChknew1/Chart ==
  state idle
    en:stat = 0;
    MdxxMemStatus=0;
  state ongoing
    en:stat = 2;
  state ispos
    en:
    stat = 1;
    MdxxMemStatus=1;
  state isposmem
    en:
    stat = 1;
    MdxxMemStatus=1;
  state InValidMem
    en:stat = 5;
  (default) -> (junction 24)
  (junction 24) -> (junction 25) [order 1] : [enflg]
  (junction 24) -> idle [order 2]
  (junction 25) -> isposmem
  idle -> ongoing [order 1] : [rsp==4]
  ongoing -> ispos [order 1] : [rsp==1]
  ongoing -> idle [order 2] : [rsp!=4]
  idle -> ispos [order 2] : [rsp==5]
  ispos -> idle : [!IsArrivedTrgtPos ]
  isposmem -> idle : [!IsArrivedTrgtPos&&after(500,tick)]
  InValidMem -> idle [order 2] : [InvalidMem ==0]
  idle -> InValidMem [order 3] : [InvalidMem ==1]
  (junction 19) -> ispos : [rsp==5]
  InValidMem -> (junction 19) [order 1] : [InvalidMem ==0]
  data: rsp input uint8; IsArrivedTrgtPos input boolean; enflg input boolean; stat output uint8; InvalidMem input boolean; MdxxMemStatus output uint32

== stateflow chart MdXX_Status/MdXX_Status_Cal_sys/Subsystem/Md6StatChknew/Chart ==
  state idle
    en:stat = 0;
    MdxxMemStatus=0;
  state ongoing
    en:stat = 2;
  state ispos
    en:
    stat = 1;
    MdxxMemStatus=1;
  state isposmem
    en:
    stat = 1;
    MdxxMemStatus=1;
  state InValidMem
    en:stat = 5;
  (default) -> (junction 24)
  (junction 24) -> (junction 25) [order 1] : [enflg]
  (junction 24) -> idle [order 2]
  (junction 25) -> isposmem
  idle -> ongoing [order 1] : [rsp==4]
  ongoing -> ispos [order 1] : [rsp==1]
  ongoing -> idle [order 2] : [rsp!=4]
  idle -> ispos [order 2] : [rsp==5]
  ispos -> idle : [!IsArrivedTrgtPos ]
  isposmem -> idle : [!IsArrivedTrgtPos&&after(500,tick)]
  InValidMem -> idle [order 2] : [InvalidMem ==0]
  idle -> InValidMem [order 3] : [InvalidMem ==1]
  (junction 19) -> ispos : [rsp==5]
  InValidMem -> (junction 19) [order 1] : [InvalidMem ==0]
  data: rsp input uint8; IsArrivedTrgtPos input boolean; enflg input boolean; stat output uint8; InvalidMem input boolean; MdxxMemStatus output uint32
